simulink model "aes_impl_decrypt_smc"  (R2015b)
settings: Solver=FixedStepDiscrete  SolverMode=SingleTasking  StartTime=0.0  StopTime=1000e-6  RelTol=1e-3
undefined symbols (not defined in the file): a, b, input_sample_rate
libraries: shlslibv1 x3018
(part 9 of 20)

== system aes_impl_decrypt_smc/Round6/Subsystem8/Subsystem2 ==
  In1 : Inport
  In2 : Inport  Port=2
  In3 : Inport  Port=3
  In4 : Inport  Port=4
  Mixcolumn : Subsystem
  Mixcolumn1 : Subsystem
  Mixcolumn2 : Subsystem
  Mixcolumn3 : Subsystem
  Out1 : Outport
  Out2 : Outport  Port=2
  Out3 : Outport  Port=3
  Out4 : Outport  Port=4
  wires:
  Mixcolumn/1(Out1) -> Out1/1
  In4/1 -> Mixcolumn/4(In4), Mixcolumn1/4(In4), Mixcolumn2/4(In4), Mixcolumn3/4(In4)
  Mixcolumn2/1(Out1) -> Out3/1
  Mixcolumn1/1(Out1) -> Out2/1
  In2/1 -> Mixcolumn/2(In2), Mixcolumn1/2(In2), Mixcolumn3/2(In2), Mixcolumn2/2(In2)
  In1/1 -> Mixcolumn2/1(In1), Mixcolumn3/1(In1), Mixcolumn1/1(In1), Mixcolumn/1(In1)
  In3/1 -> Mixcolumn/3(In3), Mixcolumn1/3(In3), Mixcolumn3/3(In3), Mixcolumn2/3(In3)
  Mixcolumn3/1(Out1) -> Out4/1

== system aes_impl_decrypt_smc/Round6/Subsystem8/Subsystem3 ==
  In1 : Inport
  In2 : Inport  Port=2
  In3 : Inport  Port=3
  In4 : Inport  Port=4
  Mixcolumn : Subsystem
  Mixcolumn1 : Subsystem
  Mixcolumn2 : Subsystem
  Mixcolumn3 : Subsystem
  Out1 : Outport
  Out2 : Outport  Port=2
  Out3 : Outport  Port=3
  Out4 : Outport  Port=4
  wires:
  Mixcolumn/1(Out1) -> Out1/1
  In4/1 -> Mixcolumn/4(In4), Mixcolumn1/4(In4), Mixcolumn2/4(In4), Mixcolumn3/4(In4)
  Mixcolumn2/1(Out1) -> Out3/1
  Mixcolumn1/1(Out1) -> Out2/1
  In2/1 -> Mixcolumn/2(In2), Mixcolumn1/2(In2), Mixcolumn3/2(In2), Mixcolumn2/2(In2)
  In1/1 -> Mixcolumn2/1(In1), Mixcolumn3/1(In1), Mixcolumn1/1(In1), Mixcolumn/1(In1)
  In3/1 -> Mixcolumn/3(In3), Mixcolumn1/3(In3), Mixcolumn3/3(In3), Mixcolumn2/3(In3)
  Mixcolumn3/1(Out1) -> Out4/1

== system aes_impl_decrypt_smc/Round6/Subsystem8/Subsystem4 ==
  In1 : Inport
  In2 : Inport  Port=2
  In3 : Inport  Port=3
  In4 : Inport  Port=4
  ROM{1..4} (4 alike) : shlslibv1/Memories/ROM  syn_rom_vec=sbox  syn_rom_auto_wl=on  syn_out_wl=8  syn_out_fl=0  syn_out_dt=unsigned  syn_out_sat=on  syn_out_rnd=on  syn_en_port=off  synBlockType=primitive  synLatency=1  synBlockId=62  syn_dual_port=off
  Out1 : Outport
  Out2 : Outport  Port=2
  Out3 : Outport  Port=3
  Out4 : Outport  Port=4
  wires:
  In1/1 -> ROM4/1
  In4/1 -> ROM3/1
  In3/1 -> ROM2/1
  ROM4/1 -> Out1/1
  ROM1/1 -> Out2/1
  ROM2/1 -> Out3/1
  ROM3/1 -> Out4/1
  In2/1 -> ROM1/1

== system aes_impl_decrypt_smc/Round6/Subsystem8/Subsystem5 ==
  In1 : Inport
  In2 : Inport  Port=2
  In3 : Inport  Port=3
  In4 : Inport  Port=4
  ROM{1..4} (4 alike) : shlslibv1/Memories/ROM  syn_rom_vec=sbox  syn_rom_auto_wl=on  syn_out_wl=8  syn_out_fl=0  syn_out_dt=unsigned  syn_out_sat=on  syn_out_rnd=on  syn_en_port=off  synBlockType=primitive  synLatency=1  synBlockId=62  syn_dual_port=off
  Out1 : Outport
  Out2 : Outport  Port=2
  Out3 : Outport  Port=3
  Out4 : Outport  Port=4
  wires:
  In1/1 -> ROM4/1
  In4/1 -> ROM3/1
  In3/1 -> ROM2/1
  ROM4/1 -> Out1/1
  ROM1/1 -> Out2/1
  ROM2/1 -> Out3/1
  ROM3/1 -> Out4/1
  In2/1 -> ROM1/1

== system aes_impl_decrypt_smc/Round6/Subsystem8/Subsystem6 ==
  In1 : Inport
  In2 : Inport  Port=2
  In3 : Inport  Port=3
  In4 : Inport  Port=4
  ROM{1..4} (4 alike) : shlslibv1/Memories/ROM  syn_rom_vec=sbox  syn_rom_auto_wl=on  syn_out_wl=8  syn_out_fl=0  syn_out_dt=unsigned  syn_out_sat=on  syn_out_rnd=on  syn_en_port=off  synBlockType=primitive  synLatency=1  synBlockId=62  syn_dual_port=off
  Out1 : Outport
  Out2 : Outport  Port=2
  Out3 : Outport  Port=3
  Out4 : Outport  Port=4
  wires:
  In1/1 -> ROM4/1
  In4/1 -> ROM3/1
  In3/1 -> ROM2/1
  ROM4/1 -> Out1/1
  ROM1/1 -> Out2/1
  ROM2/1 -> Out3/1
  ROM3/1 -> Out4/1
  In2/1 -> ROM1/1

== system aes_impl_decrypt_smc/Round6/Subsystem8/Subsystem7 ==
  In1 : Inport
  In2 : Inport  Port=2
  In3 : Inport  Port=3
  In4 : Inport  Port=4
  ROM{1..4} (4 alike) : shlslibv1/Memories/ROM  syn_rom_vec=sbox  syn_rom_auto_wl=on  syn_out_wl=8  syn_out_fl=0  syn_out_dt=unsigned  syn_out_sat=on  syn_out_rnd=on  syn_en_port=off  synBlockType=primitive  synLatency=1  synBlockId=62  syn_dual_port=off
  Out1 : Outport
  Out2 : Outport  Port=2
  Out3 : Outport  Port=3
  Out4 : Outport  Port=4
  wires:
  In1/1 -> ROM4/1
  In4/1 -> ROM3/1
  In3/1 -> ROM2/1
  ROM4/1 -> Out1/1
  ROM1/1 -> Out2/1
  ROM2/1 -> Out3/1
  ROM3/1 -> Out4/1
  In2/1 -> ROM1/1

== system aes_impl_decrypt_smc/Round7/Key1/Keygen1 ==
  In1 : Inport
  In2 : Inport  Port=2
  In3 : Inport  Port=3
  In4 : Inport  Port=4
  In5 : Inport  Port=5
  In6 : Inport  Port=6
  In7 : Inport  Port=7
  In8 : Inport  Port=8
  Binary Logic{,1..7} (8 alike) : shlslibv1/Math Functions/Binary Logic  syn_binlog_exp=a^b  synBlockType=primitive  synLatency=0  synBlockId=13
  Constant1 : shlslibv1/Sources/Constant  syn_cst_val=0  syn_cst_format=Specify  syn_cst_wl=8  syn_cst_fl=0  syn_cst_dt=unsigned  syn_cst_rnd=on  syn_cst_st=-1  synBlockType=primitive  synLatency=0  synBlockId=15
  Constant2 : shlslibv1/Sources/Constant  syn_cst_val=0  syn_cst_format=Specify  syn_cst_wl=8  syn_cst_fl=0  syn_cst_dt=unsigned  syn_cst_rnd=on  syn_cst_st=-1  synBlockType=primitive  synLatency=0  synBlockId=15
  Constant3 : shlslibv1/Sources/Constant  syn_cst_val=0  syn_cst_format=Specify  syn_cst_wl=8  syn_cst_fl=0  syn_cst_dt=unsigned  syn_cst_rnd=on  syn_cst_st=-1  synBlockType=primitive  synLatency=0  synBlockId=15
  Constant4 : shlslibv1/Sources/Constant  syn_cst_val=64  syn_cst_format=Specify  syn_cst_wl=8  syn_cst_fl=0  syn_cst_dt=unsigned  syn_cst_rnd=on  syn_cst_st=-1  synBlockType=primitive  synLatency=0  synBlockId=15
  Subsystem4 : Subsystem
  Out1 : Outport
  Out2 : Outport  Port=2
  Out3 : Outport  Port=3
  Out4 : Outport  Port=4
  wires:
  Constant1/1 -> Binary Logic3/2
  Binary Logic3/1 -> Out2/1
  Binary Logic5/1 -> Out3/1
  Binary Logic2/1 -> Out1/1
  Constant3/1 -> Binary Logic7/2
  Binary Logic7/1 -> Out4/1
  Constant2/1 -> Binary Logic5/2
  Subsystem4/3(Out3) -> Binary Logic4/2
  In7/1 -> Subsystem4/2(In2)
  In6/1 -> Subsystem4/1(In1)
  Subsystem4/4(Out4) -> Binary Logic6/2
  Subsystem4/2(Out2) -> Binary Logic1/2
  Subsystem4/1(Out1) -> Binary Logic/2
  In8/1 -> Subsystem4/3(In3)
  In5/1 -> Subsystem4/4(In4)
  In1/1 -> Binary Logic/1
  In2/1 -> Binary Logic1/1
  In3/1 -> Binary Logic4/1
  In4/1 -> Binary Logic6/1
  Constant4/1 -> Binary Logic2/2
  Binary Logic/1 -> Binary Logic2/1
  Binary Logic1/1 -> Binary Logic3/1
  Binary Logic4/1 -> Binary Logic5/1
  Binary Logic6/1 -> Binary Logic7/1

== system aes_impl_decrypt_smc/Round7/Key1/Keygen2 ==
  In1 : Inport
  In2 : Inport  Port=2
  In3 : Inport  Port=3
  In4 : Inport  Port=4
  In5 : Inport  Port=5
  In6 : Inport  Port=6
  In7 : Inport  Port=7
  In8 : Inport  Port=8
  Binary Logic{,1..3} (4 alike) : shlslibv1/Math Functions/Binary Logic  syn_binlog_exp=a^b  synBlockType=primitive  synLatency=0  synBlockId=13
  Out1 : Outport
  Out2 : Outport  Port=2
  Out3 : Outport  Port=3
  Out4 : Outport  Port=4
  wires:
  In6/1 -> Binary Logic1/2
  In2/1 -> Binary Logic1/1
  Binary Logic2/1 -> Out3/1
  In7/1 -> Binary Logic2/2
  In8/1 -> Binary Logic3/2
  Binary Logic1/1 -> Out2/1
  In3/1 -> Binary Logic2/1
  In4/1 -> Binary Logic3/1
  Binary Logic3/1 -> Out4/1
  In1/1 -> Binary Logic/1
  In5/1 -> Binary Logic/2
  Binary Logic/1 -> Out1/1

== system aes_impl_decrypt_smc/Round7/Key1/Keygen3 ==
  In1 : Inport
  In2 : Inport  Port=2
  In3 : Inport  Port=3
  In4 : Inport  Port=4
  In5 : Inport  Port=5
  In6 : Inport  Port=6
  In7 : Inport  Port=7
  In8 : Inport  Port=8
  Binary Logic{,1..3} (4 alike) : shlslibv1/Math Functions/Binary Logic  syn_binlog_exp=a^b  synBlockType=primitive  synLatency=0  synBlockId=13
  Out1 : Outport
  Out2 : Outport  Port=2
  Out3 : Outport  Port=3
  Out4 : Outport  Port=4
  wires:
  In6/1 -> Binary Logic1/2
  In2/1 -> Binary Logic1/1
  Binary Logic2/1 -> Out3/1
  In7/1 -> Binary Logic2/2
  In8/1 -> Binary Logic3/2
  Binary Logic1/1 -> Out2/1
  In3/1 -> Binary Logic2/1
  In4/1 -> Binary Logic3/1
  Binary Logic3/1 -> Out4/1
  In1/1 -> Binary Logic/1
  In5/1 -> Binary Logic/2
  Binary Logic/1 -> Out1/1

== system aes_impl_decrypt_smc/Round7/Key1/Keygen4 ==
  In1 : Inport
  In2 : Inport  Port=2
  In3 : Inport  Port=3
  In4 : Inport  Port=4
  In5 : Inport  Port=5
  In6 : Inport  Port=6
  In7 : Inport  Port=7
  In8 : Inport  Port=8
  Binary Logic{,1..3} (4 alike) : shlslibv1/Math Functions/Binary Logic  syn_binlog_exp=a^b  synBlockType=primitive  synLatency=0  synBlockId=13
  Out1 : Outport
  Out2 : Outport  Port=2
  Out3 : Outport  Port=3
  Out4 : Outport  Port=4
  wires:
  In6/1 -> Binary Logic1/2
  In2/1 -> Binary Logic1/1
  Binary Logic2/1 -> Out3/1
  In7/1 -> Binary Logic2/2
  In8/1 -> Binary Logic3/2
  Binary Logic1/1 -> Out2/1
  In3/1 -> Binary Logic2/1
  In4/1 -> Binary Logic3/1
  Binary Logic3/1 -> Out4/1
  In1/1 -> Binary Logic/1
  In5/1 -> Binary Logic/2
  Binary Logic/1 -> Out1/1

== system aes_impl_decrypt_smc/Round7/Subsystem8/Subsystem ==
  In1 : Inport
  In2 : Inport  Port=2
  In3 : Inport  Port=3
  In4 : Inport  Port=4
  Mixcolumn : Subsystem
  Mixcolumn1 : Subsystem
  Mixcolumn2 : Subsystem
  Mixcolumn3 : Subsystem
  Out1 : Outport
  Out2 : Outport  Port=2
  Out3 : Outport  Port=3
  Out4 : Outport  Port=4
  wires:
  Mixcolumn/1(Out1) -> Out1/1
  In4/1 -> Mixcolumn/4(In4), Mixcolumn1/4(In4), Mixcolumn2/4(In4), Mixcolumn3/4(In4)
  Mixcolumn2/1(Out1) -> Out3/1
  Mixcolumn1/1(Out1) -> Out2/1
  In2/1 -> Mixcolumn/2(In2), Mixcolumn1/2(In2), Mixcolumn3/2(In2), Mixcolumn2/2(In2)
  In1/1 -> Mixcolumn2/1(In1), Mixcolumn3/1(In1), Mixcolumn1/1(In1), Mixcolumn/1(In1)
  In3/1 -> Mixcolumn/3(In3), Mixcolumn1/3(In3), Mixcolumn3/3(In3), Mixcolumn2/3(In3)
  Mixcolumn3/1(Out1) -> Out4/1

== system aes_impl_decrypt_smc/Round7/Subsystem8/Subsystem1 ==
  In1 : Inport
  In2 : Inport  Port=2
  In3 : Inport  Port=3
  In4 : Inport  Port=4
  Mixcolumn : Subsystem
  Mixcolumn1 : Subsystem
  Mixcolumn2 : Subsystem
  Mixcolumn3 : Subsystem
  Out1 : Outport
  Out2 : Outport  Port=2
  Out3 : Outport  Port=3
  Out4 : Outport  Port=4
  wires:
  Mixcolumn/1(Out1) -> Out1/1
  In4/1 -> Mixcolumn/4(In4), Mixcolumn1/4(In4), Mixcolumn2/4(In4), Mixcolumn3/4(In4)
  Mixcolumn2/1(Out1) -> Out3/1
  Mixcolumn1/1(Out1) -> Out2/1
  In2/1 -> Mixcolumn/2(In2), Mixcolumn1/2(In2), Mixcolumn3/2(In2), Mixcolumn2/2(In2)
  In1/1 -> Mixcolumn2/1(In1), Mixcolumn3/1(In1), Mixcolumn1/1(In1), Mixcolumn/1(In1)
  In3/1 -> Mixcolumn/3(In3), Mixcolumn1/3(In3), Mixcolumn3/3(In3), Mixcolumn2/3(In3)
  Mixcolumn3/1(Out1) -> Out4/1

== system aes_impl_decrypt_smc/Round7/Subsystem8/Subsystem2 ==
  In1 : Inport
  In2 : Inport  Port=2
  In3 : Inport  Port=3
  In4 : Inport  Port=4
  Mixcolumn : Subsystem
  Mixcolumn1 : Subsystem
  Mixcolumn2 : Subsystem
  Mixcolumn3 : Subsystem
  Out1 : Outport
  Out2 : Outport  Port=2
  Out3 : Outport  Port=3
  Out4 : Outport  Port=4
  wires:
  Mixcolumn/1(Out1) -> Out1/1
  In4/1 -> Mixcolumn/4(In4), Mixcolumn1/4(In4), Mixcolumn2/4(In4), Mixcolumn3/4(In4)
  Mixcolumn2/1(Out1) -> Out3/1
  Mixcolumn1/1(Out1) -> Out2/1
  In2/1 -> Mixcolumn/2(In2), Mixcolumn1/2(In2), Mixcolumn3/2(In2), Mixcolumn2/2(In2)
  In1/1 -> Mixcolumn2/1(In1), Mixcolumn3/1(In1), Mixcolumn1/1(In1), Mixcolumn/1(In1)
  In3/1 -> Mixcolumn/3(In3), Mixcolumn1/3(In3), Mixcolumn3/3(In3), Mixcolumn2/3(In3)
  Mixcolumn3/1(Out1) -> Out4/1

== system aes_impl_decrypt_smc/Round7/Subsystem8/Subsystem3 ==
  In1 : Inport
  In2 : Inport  Port=2
  In3 : Inport  Port=3
  In4 : Inport  Port=4
  Mixcolumn : Subsystem
  Mixcolumn1 : Subsystem
  Mixcolumn2 : Subsystem
  Mixcolumn3 : Subsystem
  Out1 : Outport
  Out2 : Outport  Port=2
  Out3 : Outport  Port=3
  Out4 : Outport  Port=4
  wires:
  Mixcolumn/1(Out1) -> Out1/1
  In4/1 -> Mixcolumn/4(In4), Mixcolumn1/4(In4), Mixcolumn2/4(In4), Mixcolumn3/4(In4)
  Mixcolumn2/1(Out1) -> Out3/1
  Mixcolumn1/1(Out1) -> Out2/1
  In2/1 -> Mixcolumn/2(In2), Mixcolumn1/2(In2), Mixcolumn3/2(In2), Mixcolumn2/2(In2)
  In1/1 -> Mixcolumn2/1(In1), Mixcolumn3/1(In1), Mixcolumn1/1(In1), Mixcolumn/1(In1)
  In3/1 -> Mixcolumn/3(In3), Mixcolumn1/3(In3), Mixcolumn3/3(In3), Mixcolumn2/3(In3)
  Mixcolumn3/1(Out1) -> Out4/1

== system aes_impl_decrypt_smc/Round7/Subsystem8/Subsystem4 ==
  In1 : Inport
  In2 : Inport  Port=2
  In3 : Inport  Port=3
  In4 : Inport  Port=4
  ROM{1..4} (4 alike) : shlslibv1/Memories/ROM  syn_rom_vec=sbox  syn_rom_auto_wl=on  syn_out_wl=8  syn_out_fl=0  syn_out_dt=unsigned  syn_out_sat=on  syn_out_rnd=on  syn_en_port=off  synBlockType=primitive  synLatency=1  synBlockId=62  syn_dual_port=off
  Out1 : Outport
  Out2 : Outport  Port=2
  Out3 : Outport  Port=3
  Out4 : Outport  Port=4
  wires:
  In1/1 -> ROM4/1
  In4/1 -> ROM3/1
  In3/1 -> ROM2/1
  ROM4/1 -> Out1/1
  ROM1/1 -> Out2/1
  ROM2/1 -> Out3/1
  ROM3/1 -> Out4/1
  In2/1 -> ROM1/1

== system aes_impl_decrypt_smc/Round7/Subsystem8/Subsystem5 ==
  In1 : Inport
  In2 : Inport  Port=2
  In3 : Inport  Port=3
  In4 : Inport  Port=4
  ROM{1..4} (4 alike) : shlslibv1/Memories/ROM  syn_rom_vec=sbox  syn_rom_auto_wl=on  syn_out_wl=8  syn_out_fl=0  syn_out_dt=unsigned  syn_out_sat=on  syn_out_rnd=on  syn_en_port=off  synBlockType=primitive  synLatency=1  synBlockId=62  syn_dual_port=off
  Out1 : Outport
  Out2 : Outport  Port=2
  Out3 : Outport  Port=3
  Out4 : Outport  Port=4
  wires:
  In1/1 -> ROM4/1
  In4/1 -> ROM3/1
  In3/1 -> ROM2/1
  ROM4/1 -> Out1/1
  ROM1/1 -> Out2/1
  ROM2/1 -> Out3/1
  ROM3/1 -> Out4/1
  In2/1 -> ROM1/1

== system aes_impl_decrypt_smc/Round7/Subsystem8/Subsystem6 ==
  In1 : Inport
  In2 : Inport  Port=2
  In3 : Inport  Port=3
  In4 : Inport  Port=4
  ROM{1..4} (4 alike) : shlslibv1/Memories/ROM  syn_rom_vec=sbox  syn_rom_auto_wl=on  syn_out_wl=8  syn_out_fl=0  syn_out_dt=unsigned  syn_out_sat=on  syn_out_rnd=on  syn_en_port=off  synBlockType=primitive  synLatency=1  synBlockId=62  syn_dual_port=off
  Out1 : Outport
  Out2 : Outport  Port=2
  Out3 : Outport  Port=3
  Out4 : Outport  Port=4
  wires:
  In1/1 -> ROM4/1
  In4/1 -> ROM3/1
  In3/1 -> ROM2/1
  ROM4/1 -> Out1/1
  ROM1/1 -> Out2/1
  ROM2/1 -> Out3/1
  ROM3/1 -> Out4/1
  In2/1 -> ROM1/1

== system aes_impl_decrypt_smc/Round7/Subsystem8/Subsystem7 ==
  In1 : Inport
  In2 : Inport  Port=2
  In3 : Inport  Port=3
  In4 : Inport  Port=4
  ROM{1..4} (4 alike) : shlslibv1/Memories/ROM  syn_rom_vec=sbox  syn_rom_auto_wl=on  syn_out_wl=8  syn_out_fl=0  syn_out_dt=unsigned  syn_out_sat=on  syn_out_rnd=on  syn_en_port=off  synBlockType=primitive  synLatency=1  synBlockId=62  syn_dual_port=off
  Out1 : Outport
  Out2 : Outport  Port=2
  Out3 : Outport  Port=3
  Out4 : Outport  Port=4
  wires:
  In1/1 -> ROM4/1
  In4/1 -> ROM3/1
  In3/1 -> ROM2/1
  ROM4/1 -> Out1/1
  ROM1/1 -> Out2/1
  ROM2/1 -> Out3/1
  ROM3/1 -> Out4/1
  In2/1 -> ROM1/1

== system aes_impl_decrypt_smc/Round8/Key1/Keygen1 ==
  In1 : Inport
  In2 : Inport  Port=2
  In3 : Inport  Port=3
  In4 : Inport  Port=4
  In5 : Inport  Port=5
  In6 : Inport  Port=6
  In7 : Inport  Port=7
  In8 : Inport  Port=8
  Binary Logic{,1..7} (8 alike) : shlslibv1/Math Functions/Binary Logic  syn_binlog_exp=a^b  synBlockType=primitive  synLatency=0  synBlockId=13
  Constant1 : shlslibv1/Sources/Constant  syn_cst_val=0  syn_cst_format=Specify  syn_cst_wl=8  syn_cst_fl=0  syn_cst_dt=unsigned  syn_cst_rnd=on  syn_cst_st=-1  synBlockType=primitive  synLatency=0  synBlockId=15
  Constant2 : shlslibv1/Sources/Constant  syn_cst_val=0  syn_cst_format=Specify  syn_cst_wl=8  syn_cst_fl=0  syn_cst_dt=unsigned  syn_cst_rnd=on  syn_cst_st=-1  synBlockType=primitive  synLatency=0  synBlockId=15
  Constant3 : shlslibv1/Sources/Constant  syn_cst_val=0  syn_cst_format=Specify  syn_cst_wl=8  syn_cst_fl=0  syn_cst_dt=unsigned  syn_cst_rnd=on  syn_cst_st=-1  synBlockType=primitive  synLatency=0  synBlockId=15
  Constant4 : shlslibv1/Sources/Constant  syn_cst_val=128  syn_cst_format=Specify  syn_cst_wl=8  syn_cst_fl=0  syn_cst_dt=unsigned  syn_cst_rnd=on  syn_cst_st=-1  synBlockType=primitive  synLatency=0  synBlockId=15
  Subsystem4 : Subsystem
  Out1 : Outport
  Out2 : Outport  Port=2
  Out3 : Outport  Port=3
  Out4 : Outport  Port=4
  wires:
  Constant1/1 -> Binary Logic3/2
  Binary Logic3/1 -> Out2/1
  Binary Logic5/1 -> Out3/1
  Binary Logic2/1 -> Out1/1
  Constant3/1 -> Binary Logic7/2
  Binary Logic7/1 -> Out4/1
  Constant2/1 -> Binary Logic5/2
  Subsystem4/3(Out3) -> Binary Logic4/2
  In7/1 -> Subsystem4/2(In2)
  In6/1 -> Subsystem4/1(In1)
  Subsystem4/4(Out4) -> Binary Logic6/2
  Subsystem4/2(Out2) -> Binary Logic1/2
  Subsystem4/1(Out1) -> Binary Logic/2
  In8/1 -> Subsystem4/3(In3)
  In5/1 -> Subsystem4/4(In4)
  In1/1 -> Binary Logic/1
  In2/1 -> Binary Logic1/1
  In3/1 -> Binary Logic4/1
  In4/1 -> Binary Logic6/1
  Constant4/1 -> Binary Logic2/2
  Binary Logic/1 -> Binary Logic2/1
  Binary Logic1/1 -> Binary Logic3/1
  Binary Logic4/1 -> Binary Logic5/1
  Binary Logic6/1 -> Binary Logic7/1

== system aes_impl_decrypt_smc/Round8/Key1/Keygen2 ==
  In1 : Inport
  In2 : Inport  Port=2
  In3 : Inport  Port=3
  In4 : Inport  Port=4
  In5 : Inport  Port=5
  In6 : Inport  Port=6
  In7 : Inport  Port=7
  In8 : Inport  Port=8
  Binary Logic{,1..3} (4 alike) : shlslibv1/Math Functions/Binary Logic  syn_binlog_exp=a^b  synBlockType=primitive  synLatency=0  synBlockId=13
  Out1 : Outport
  Out2 : Outport  Port=2
  Out3 : Outport  Port=3
  Out4 : Outport  Port=4
  wires:
  In6/1 -> Binary Logic1/2
  In2/1 -> Binary Logic1/1
  Binary Logic2/1 -> Out3/1
  In7/1 -> Binary Logic2/2
  In8/1 -> Binary Logic3/2
  Binary Logic1/1 -> Out2/1
  In3/1 -> Binary Logic2/1
  In4/1 -> Binary Logic3/1
  Binary Logic3/1 -> Out4/1
  In1/1 -> Binary Logic/1
  In5/1 -> Binary Logic/2
  Binary Logic/1 -> Out1/1

== system aes_impl_decrypt_smc/Round8/Key1/Keygen3 ==
  In1 : Inport
  In2 : Inport  Port=2
  In3 : Inport  Port=3
  In4 : Inport  Port=4
  In5 : Inport  Port=5
  In6 : Inport  Port=6
  In7 : Inport  Port=7
  In8 : Inport  Port=8
  Binary Logic{,1..3} (4 alike) : shlslibv1/Math Functions/Binary Logic  syn_binlog_exp=a^b  synBlockType=primitive  synLatency=0  synBlockId=13
  Out1 : Outport
  Out2 : Outport  Port=2
  Out3 : Outport  Port=3
  Out4 : Outport  Port=4
  wires:
  In6/1 -> Binary Logic1/2
  In2/1 -> Binary Logic1/1
  Binary Logic2/1 -> Out3/1
  In7/1 -> Binary Logic2/2
  In8/1 -> Binary Logic3/2
  Binary Logic1/1 -> Out2/1
  In3/1 -> Binary Logic2/1
  In4/1 -> Binary Logic3/1
  Binary Logic3/1 -> Out4/1
  In1/1 -> Binary Logic/1
  In5/1 -> Binary Logic/2
  Binary Logic/1 -> Out1/1

== system aes_impl_decrypt_smc/Round8/Key1/Keygen4 ==
  In1 : Inport
  In2 : Inport  Port=2
  In3 : Inport  Port=3
  In4 : Inport  Port=4
  In5 : Inport  Port=5
  In6 : Inport  Port=6
  In7 : Inport  Port=7
  In8 : Inport  Port=8
  Binary Logic{,1..3} (4 alike) : shlslibv1/Math Functions/Binary Logic  syn_binlog_exp=a^b  synBlockType=primitive  synLatency=0  synBlockId=13
  Out1 : Outport
  Out2 : Outport  Port=2
  Out3 : Outport  Port=3
  Out4 : Outport  Port=4
  wires:
  In6/1 -> Binary Logic1/2
  In2/1 -> Binary Logic1/1
  Binary Logic2/1 -> Out3/1
  In7/1 -> Binary Logic2/2
  In8/1 -> Binary Logic3/2
  Binary Logic1/1 -> Out2/1
  In3/1 -> Binary Logic2/1
  In4/1 -> Binary Logic3/1
  Binary Logic3/1 -> Out4/1
  In1/1 -> Binary Logic/1
  In5/1 -> Binary Logic/2
  Binary Logic/1 -> Out1/1

== system aes_impl_decrypt_smc/Round8/Subsystem8/Subsystem ==
  In1 : Inport
  In2 : Inport  Port=2
  In3 : Inport  Port=3
  In4 : Inport  Port=4
  Mixcolumn : Subsystem
  Mixcolumn1 : Subsystem
  Mixcolumn2 : Subsystem
  Mixcolumn3 : Subsystem
  Out1 : Outport
  Out2 : Outport  Port=2
  Out3 : Outport  Port=3
  Out4 : Outport  Port=4
  wires:
  Mixcolumn/1(Out1) -> Out1/1
  In4/1 -> Mixcolumn/4(In4), Mixcolumn1/4(In4), Mixcolumn2/4(In4), Mixcolumn3/4(In4)
  Mixcolumn2/1(Out1) -> Out3/1
  Mixcolumn1/1(Out1) -> Out2/1
  In2/1 -> Mixcolumn/2(In2), Mixcolumn1/2(In2), Mixcolumn3/2(In2), Mixcolumn2/2(In2)
  In1/1 -> Mixcolumn2/1(In1), Mixcolumn3/1(In1), Mixcolumn1/1(In1), Mixcolumn/1(In1)
  In3/1 -> Mixcolumn/3(In3), Mixcolumn1/3(In3), Mixcolumn3/3(In3), Mixcolumn2/3(In3)
  Mixcolumn3/1(Out1) -> Out4/1

== system aes_impl_decrypt_smc/Round8/Subsystem8/Subsystem1 ==
  In1 : Inport
  In2 : Inport  Port=2
  In3 : Inport  Port=3
  In4 : Inport  Port=4
  Mixcolumn : Subsystem
  Mixcolumn1 : Subsystem
  Mixcolumn2 : Subsystem
  Mixcolumn3 : Subsystem
  Out1 : Outport
  Out2 : Outport  Port=2
  Out3 : Outport  Port=3
  Out4 : Outport  Port=4
  wires:
  Mixcolumn/1(Out1) -> Out1/1
  In4/1 -> Mixcolumn/4(In4), Mixcolumn1/4(In4), Mixcolumn2/4(In4), Mixcolumn3/4(In4)
  Mixcolumn2/1(Out1) -> Out3/1
  Mixcolumn1/1(Out1) -> Out2/1
  In2/1 -> Mixcolumn/2(In2), Mixcolumn1/2(In2), Mixcolumn3/2(In2), Mixcolumn2/2(In2)
  In1/1 -> Mixcolumn2/1(In1), Mixcolumn3/1(In1), Mixcolumn1/1(In1), Mixcolumn/1(In1)
  In3/1 -> Mixcolumn/3(In3), Mixcolumn1/3(In3), Mixcolumn3/3(In3), Mixcolumn2/3(In3)
  Mixcolumn3/1(Out1) -> Out4/1

== system aes_impl_decrypt_smc/Round8/Subsystem8/Subsystem2 ==
  In1 : Inport
  In2 : Inport  Port=2
  In3 : Inport  Port=3
  In4 : Inport  Port=4
  Mixcolumn : Subsystem
  Mixcolumn1 : Subsystem
  Mixcolumn2 : Subsystem
  Mixcolumn3 : Subsystem
  Out1 : Outport
  Out2 : Outport  Port=2
  Out3 : Outport  Port=3
  Out4 : Outport  Port=4
  wires:
  Mixcolumn/1(Out1) -> Out1/1
  In4/1 -> Mixcolumn/4(In4), Mixcolumn1/4(In4), Mixcolumn2/4(In4), Mixcolumn3/4(In4)
  Mixcolumn2/1(Out1) -> Out3/1
  Mixcolumn1/1(Out1) -> Out2/1
  In2/1 -> Mixcolumn/2(In2), Mixcolumn1/2(In2), Mixcolumn3/2(In2), Mixcolumn2/2(In2)
  In1/1 -> Mixcolumn2/1(In1), Mixcolumn3/1(In1), Mixcolumn1/1(In1), Mixcolumn/1(In1)
  In3/1 -> Mixcolumn/3(In3), Mixcolumn1/3(In3), Mixcolumn3/3(In3), Mixcolumn2/3(In3)
  Mixcolumn3/1(Out1) -> Out4/1

== system aes_impl_decrypt_smc/Round8/Subsystem8/Subsystem3 ==
  In1 : Inport
  In2 : Inport  Port=2
  In3 : Inport  Port=3
  In4 : Inport  Port=4
  Mixcolumn : Subsystem
  Mixcolumn1 : Subsystem
  Mixcolumn2 : Subsystem
  Mixcolumn3 : Subsystem
  Out1 : Outport
  Out2 : Outport  Port=2
  Out3 : Outport  Port=3
  Out4 : Outport  Port=4
  wires:
  Mixcolumn/1(Out1) -> Out1/1
  In4/1 -> Mixcolumn/4(In4), Mixcolumn1/4(In4), Mixcolumn2/4(In4), Mixcolumn3/4(In4)
  Mixcolumn2/1(Out1) -> Out3/1
  Mixcolumn1/1(Out1) -> Out2/1
  In2/1 -> Mixcolumn/2(In2), Mixcolumn1/2(In2), Mixcolumn3/2(In2), Mixcolumn2/2(In2)
  In1/1 -> Mixcolumn2/1(In1), Mixcolumn3/1(In1), Mixcolumn1/1(In1), Mixcolumn/1(In1)
  In3/1 -> Mixcolumn/3(In3), Mixcolumn1/3(In3), Mixcolumn3/3(In3), Mixcolumn2/3(In3)
  Mixcolumn3/1(Out1) -> Out4/1

== system aes_impl_decrypt_smc/Round8/Subsystem8/Subsystem4 ==
  In1 : Inport
  In2 : Inport  Port=2
  In3 : Inport  Port=3
  In4 : Inport  Port=4
  ROM{1..4} (4 alike) : shlslibv1/Memories/ROM  syn_rom_vec=sbox  syn_rom_auto_wl=on  syn_out_wl=8  syn_out_fl=0  syn_out_dt=unsigned  syn_out_sat=on  syn_out_rnd=on  syn_en_port=off  synBlockType=primitive  synLatency=1  synBlockId=62  syn_dual_port=off
  Out1 : Outport
  Out2 : Outport  Port=2
  Out3 : Outport  Port=3
  Out4 : Outport  Port=4
  wires:
  In1/1 -> ROM4/1
  In4/1 -> ROM3/1
  In3/1 -> ROM2/1
  ROM4/1 -> Out1/1
  ROM1/1 -> Out2/1
  ROM2/1 -> Out3/1
  ROM3/1 -> Out4/1
  In2/1 -> ROM1/1

== system aes_impl_decrypt_smc/Round8/Subsystem8/Subsystem5 ==
  In1 : Inport
  In2 : Inport  Port=2
  In3 : Inport  Port=3
  In4 : Inport  Port=4
  ROM{1..4} (4 alike) : shlslibv1/Memories/ROM  syn_rom_vec=sbox  syn_rom_auto_wl=on  syn_out_wl=8  syn_out_fl=0  syn_out_dt=unsigned  syn_out_sat=on  syn_out_rnd=on  syn_en_port=off  synBlockType=primitive  synLatency=1  synBlockId=62  syn_dual_port=off
  Out1 : Outport
  Out2 : Outport  Port=2
  Out3 : Outport  Port=3
  Out4 : Outport  Port=4
  wires:
  In1/1 -> ROM4/1
  In4/1 -> ROM3/1
  In3/1 -> ROM2/1
  ROM4/1 -> Out1/1
  ROM1/1 -> Out2/1
  ROM2/1 -> Out3/1
  ROM3/1 -> Out4/1
  In2/1 -> ROM1/1

== system aes_impl_decrypt_smc/Round8/Subsystem8/Subsystem6 ==
  In1 : Inport
  In2 : Inport  Port=2
  In3 : Inport  Port=3
  In4 : Inport  Port=4
  ROM{1..4} (4 alike) : shlslibv1/Memories/ROM  syn_rom_vec=sbox  syn_rom_auto_wl=on  syn_out_wl=8  syn_out_fl=0  syn_out_dt=unsigned  syn_out_sat=on  syn_out_rnd=on  syn_en_port=off  synBlockType=primitive  synLatency=1  synBlockId=62  syn_dual_port=off
  Out1 : Outport
  Out2 : Outport  Port=2
  Out3 : Outport  Port=3
  Out4 : Outport  Port=4
  wires:
  In1/1 -> ROM4/1
  In4/1 -> ROM3/1
  In3/1 -> ROM2/1
  ROM4/1 -> Out1/1
  ROM1/1 -> Out2/1
  ROM2/1 -> Out3/1
  ROM3/1 -> Out4/1
  In2/1 -> ROM1/1

== system aes_impl_decrypt_smc/Round8/Subsystem8/Subsystem7 ==
  In1 : Inport
  In2 : Inport  Port=2
  In3 : Inport  Port=3
  In4 : Inport  Port=4
  ROM{1..4} (4 alike) : shlslibv1/Memories/ROM  syn_rom_vec=sbox  syn_rom_auto_wl=on  syn_out_wl=8  syn_out_fl=0  syn_out_dt=unsigned  syn_out_sat=on  syn_out_rnd=on  syn_en_port=off  synBlockType=primitive  synLatency=1  synBlockId=62  syn_dual_port=off
  Out1 : Outport
  Out2 : Outport  Port=2
  Out3 : Outport  Port=3
  Out4 : Outport  Port=4
  wires:
  In1/1 -> ROM4/1
  In4/1 -> ROM3/1
  In3/1 -> ROM2/1
  ROM4/1 -> Out1/1
  ROM1/1 -> Out2/1
  ROM2/1 -> Out3/1
  ROM3/1 -> Out4/1
  In2/1 -> ROM1/1

== system aes_impl_decrypt_smc/Round9/Key1/Keygen1 ==
  In1 : Inport
  In2 : Inport  Port=2
  In3 : Inport  Port=3
  In4 : Inport  Port=4
  In5 : Inport  Port=5
  In6 : Inport  Port=6
  In7 : Inport  Port=7
  In8 : Inport  Port=8
  Binary Logic{,1..7} (8 alike) : shlslibv1/Math Functions/Binary Logic  syn_binlog_exp=a^b  synBlockType=primitive  synLatency=0  synBlockId=13
  Constant1 : shlslibv1/Sources/Constant  syn_cst_val=0  syn_cst_format=Specify  syn_cst_wl=8  syn_cst_fl=0  syn_cst_dt=unsigned  syn_cst_rnd=on  syn_cst_st=-1  synBlockType=primitive  synLatency=0  synBlockId=15
  Constant2 : shlslibv1/Sources/Constant  syn_cst_val=0  syn_cst_format=Specify  syn_cst_wl=8  syn_cst_fl=0  syn_cst_dt=unsigned  syn_cst_rnd=on  syn_cst_st=-1  synBlockType=primitive  synLatency=0  synBlockId=15
  Constant3 : shlslibv1/Sources/Constant  syn_cst_val=0  syn_cst_format=Specify  syn_cst_wl=8  syn_cst_fl=0  syn_cst_dt=unsigned  syn_cst_rnd=on  syn_cst_st=-1  synBlockType=primitive  synLatency=0  synBlockId=15
  Constant4 : shlslibv1/Sources/Constant  syn_cst_val=27  syn_cst_format=Specify  syn_cst_wl=8  syn_cst_fl=0  syn_cst_dt=unsigned  syn_cst_rnd=on  syn_cst_st=-1  synBlockType=primitive  synLatency=0  synBlockId=15
  Subsystem4 : Subsystem
  Out1 : Outport
  Out2 : Outport  Port=2
  Out3 : Outport  Port=3
  Out4 : Outport  Port=4
  wires:
  Constant1/1 -> Binary Logic3/2
  Binary Logic3/1 -> Out2/1
  Binary Logic5/1 -> Out3/1
  Binary Logic2/1 -> Out1/1
  Constant3/1 -> Binary Logic7/2
  Binary Logic7/1 -> Out4/1
  Constant2/1 -> Binary Logic5/2
  Subsystem4/3(Out3) -> Binary Logic4/2
  In7/1 -> Subsystem4/2(In2)
  In6/1 -> Subsystem4/1(In1)
  Subsystem4/4(Out4) -> Binary Logic6/2
  Subsystem4/2(Out2) -> Binary Logic1/2
  Subsystem4/1(Out1) -> Binary Logic/2
  In8/1 -> Subsystem4/3(In3)
  In5/1 -> Subsystem4/4(In4)
  In1/1 -> Binary Logic/1
  In2/1 -> Binary Logic1/1
  In3/1 -> Binary Logic4/1
  In4/1 -> Binary Logic6/1
  Constant4/1 -> Binary Logic2/2
  Binary Logic/1 -> Binary Logic2/1
  Binary Logic1/1 -> Binary Logic3/1
  Binary Logic4/1 -> Binary Logic5/1
  Binary Logic6/1 -> Binary Logic7/1

== system aes_impl_decrypt_smc/Round9/Key1/Keygen2 ==
  In1 : Inport
  In2 : Inport  Port=2
  In3 : Inport  Port=3
  In4 : Inport  Port=4
  In5 : Inport  Port=5
  In6 : Inport  Port=6
  In7 : Inport  Port=7
  In8 : Inport  Port=8
  Binary Logic{,1..3} (4 alike) : shlslibv1/Math Functions/Binary Logic  syn_binlog_exp=a^b  synBlockType=primitive  synLatency=0  synBlockId=13
  Out1 : Outport
  Out2 : Outport  Port=2
  Out3 : Outport  Port=3
  Out4 : Outport  Port=4
  wires:
  In6/1 -> Binary Logic1/2
  In2/1 -> Binary Logic1/1
  Binary Logic2/1 -> Out3/1
  In7/1 -> Binary Logic2/2
  In8/1 -> Binary Logic3/2
  Binary Logic1/1 -> Out2/1
  In3/1 -> Binary Logic2/1
  In4/1 -> Binary Logic3/1
  Binary Logic3/1 -> Out4/1
  In1/1 -> Binary Logic/1
  In5/1 -> Binary Logic/2
  Binary Logic/1 -> Out1/1

== system aes_impl_decrypt_smc/Round9/Key1/Keygen3 ==
  In1 : Inport
  In2 : Inport  Port=2
  In3 : Inport  Port=3
  In4 : Inport  Port=4
  In5 : Inport  Port=5
  In6 : Inport  Port=6
  In7 : Inport  Port=7
  In8 : Inport  Port=8
  Binary Logic{,1..3} (4 alike) : shlslibv1/Math Functions/Binary Logic  syn_binlog_exp=a^b  synBlockType=primitive  synLatency=0  synBlockId=13
  Out1 : Outport
  Out2 : Outport  Port=2
  Out3 : Outport  Port=3
  Out4 : Outport  Port=4
  wires:
  In6/1 -> Binary Logic1/2
  In2/1 -> Binary Logic1/1
  Binary Logic2/1 -> Out3/1
  In7/1 -> Binary Logic2/2
  In8/1 -> Binary Logic3/2
  Binary Logic1/1 -> Out2/1
  In3/1 -> Binary Logic2/1
  In4/1 -> Binary Logic3/1
  Binary Logic3/1 -> Out4/1
  In1/1 -> Binary Logic/1
  In5/1 -> Binary Logic/2
  Binary Logic/1 -> Out1/1

== system aes_impl_decrypt_smc/Round9/Key1/Keygen4 ==
  In1 : Inport
  In2 : Inport  Port=2
  In3 : Inport  Port=3
  In4 : Inport  Port=4
  In5 : Inport  Port=5
  In6 : Inport  Port=6
  In7 : Inport  Port=7
  In8 : Inport  Port=8
  Binary Logic{,1..3} (4 alike) : shlslibv1/Math Functions/Binary Logic  syn_binlog_exp=a^b  synBlockType=primitive  synLatency=0  synBlockId=13
  Out1 : Outport
  Out2 : Outport  Port=2
  Out3 : Outport  Port=3
  Out4 : Outport  Port=4
  wires:
  In6/1 -> Binary Logic1/2
  In2/1 -> Binary Logic1/1
  Binary Logic2/1 -> Out3/1
  In7/1 -> Binary Logic2/2
  In8/1 -> Binary Logic3/2
  Binary Logic1/1 -> Out2/1
  In3/1 -> Binary Logic2/1
  In4/1 -> Binary Logic3/1
  Binary Logic3/1 -> Out4/1
  In1/1 -> Binary Logic/1
  In5/1 -> Binary Logic/2
  Binary Logic/1 -> Out1/1

== system aes_impl_decrypt_smc/Round9/Subsystem8/Subsystem ==
  In1 : Inport
  In2 : Inport  Port=2
  In3 : Inport  Port=3
  In4 : Inport  Port=4
  Mixcolumn : Subsystem
  Mixcolumn1 : Subsystem
  Mixcolumn2 : Subsystem
  Mixcolumn3 : Subsystem
  Out1 : Outport
  Out2 : Outport  Port=2
  Out3 : Outport  Port=3
  Out4 : Outport  Port=4
  wires:
  Mixcolumn/1(Out1) -> Out1/1
  In4/1 -> Mixcolumn/4(In4), Mixcolumn1/4(In4), Mixcolumn2/4(In4), Mixcolumn3/4(In4)
  Mixcolumn2/1(Out1) -> Out3/1
  Mixcolumn1/1(Out1) -> Out2/1
  In2/1 -> Mixcolumn/2(In2), Mixcolumn1/2(In2), Mixcolumn3/2(In2), Mixcolumn2/2(In2)
  In1/1 -> Mixcolumn2/1(In1), Mixcolumn3/1(In1), Mixcolumn1/1(In1), Mixcolumn/1(In1)
  In3/1 -> Mixcolumn/3(In3), Mixcolumn1/3(In3), Mixcolumn3/3(In3), Mixcolumn2/3(In3)
  Mixcolumn3/1(Out1) -> Out4/1

== system aes_impl_decrypt_smc/Round9/Subsystem8/Subsystem1 ==
  In1 : Inport
  In2 : Inport  Port=2
  In3 : Inport  Port=3
  In4 : Inport  Port=4
  Mixcolumn : Subsystem
  Mixcolumn1 : Subsystem
  Mixcolumn2 : Subsystem
  Mixcolumn3 : Subsystem
  Out1 : Outport
  Out2 : Outport  Port=2
  Out3 : Outport  Port=3
  Out4 : Outport  Port=4
  wires:
  Mixcolumn/1(Out1) -> Out1/1
  In4/1 -> Mixcolumn/4(In4), Mixcolumn1/4(In4), Mixcolumn2/4(In4), Mixcolumn3/4(In4)
  Mixcolumn2/1(Out1) -> Out3/1
  Mixcolumn1/1(Out1) -> Out2/1
  In2/1 -> Mixcolumn/2(In2), Mixcolumn1/2(In2), Mixcolumn3/2(In2), Mixcolumn2/2(In2)
  In1/1 -> Mixcolumn2/1(In1), Mixcolumn3/1(In1), Mixcolumn1/1(In1), Mixcolumn/1(In1)
  In3/1 -> Mixcolumn/3(In3), Mixcolumn1/3(In3), Mixcolumn3/3(In3), Mixcolumn2/3(In3)
  Mixcolumn3/1(Out1) -> Out4/1

== system aes_impl_decrypt_smc/Round9/Subsystem8/Subsystem2 ==
  In1 : Inport
  In2 : Inport  Port=2
  In3 : Inport  Port=3
  In4 : Inport  Port=4
  Mixcolumn : Subsystem
  Mixcolumn1 : Subsystem
  Mixcolumn2 : Subsystem
  Mixcolumn3 : Subsystem
  Out1 : Outport
  Out2 : Outport  Port=2
  Out3 : Outport  Port=3
  Out4 : Outport  Port=4
  wires:
  Mixcolumn/1(Out1) -> Out1/1
  In4/1 -> Mixcolumn/4(In4), Mixcolumn1/4(In4), Mixcolumn2/4(In4), Mixcolumn3/4(In4)
  Mixcolumn2/1(Out1) -> Out3/1
  Mixcolumn1/1(Out1) -> Out2/1
  In2/1 -> Mixcolumn/2(In2), Mixcolumn1/2(In2), Mixcolumn3/2(In2), Mixcolumn2/2(In2)
  In1/1 -> Mixcolumn2/1(In1), Mixcolumn3/1(In1), Mixcolumn1/1(In1), Mixcolumn/1(In1)
  In3/1 -> Mixcolumn/3(In3), Mixcolumn1/3(In3), Mixcolumn3/3(In3), Mixcolumn2/3(In3)
  Mixcolumn3/1(Out1) -> Out4/1

== system aes_impl_decrypt_smc/Round9/Subsystem8/Subsystem3 ==
  In1 : Inport
  In2 : Inport  Port=2
  In3 : Inport  Port=3
  In4 : Inport  Port=4
  Mixcolumn : Subsystem
  Mixcolumn1 : Subsystem
  Mixcolumn2 : Subsystem
  Mixcolumn3 : Subsystem
  Out1 : Outport
  Out2 : Outport  Port=2
  Out3 : Outport  Port=3
  Out4 : Outport  Port=4
  wires:
  Mixcolumn/1(Out1) -> Out1/1
  In4/1 -> Mixcolumn/4(In4), Mixcolumn1/4(In4), Mixcolumn2/4(In4), Mixcolumn3/4(In4)
  Mixcolumn2/1(Out1) -> Out3/1
  Mixcolumn1/1(Out1) -> Out2/1
  In2/1 -> Mixcolumn/2(In2), Mixcolumn1/2(In2), Mixcolumn3/2(In2), Mixcolumn2/2(In2)
  In1/1 -> Mixcolumn2/1(In1), Mixcolumn3/1(In1), Mixcolumn1/1(In1), Mixcolumn/1(In1)
  In3/1 -> Mixcolumn/3(In3), Mixcolumn1/3(In3), Mixcolumn3/3(In3), Mixcolumn2/3(In3)
  Mixcolumn3/1(Out1) -> Out4/1

== system aes_impl_decrypt_smc/Round9/Subsystem8/Subsystem4 ==
  In1 : Inport
  In2 : Inport  Port=2
  In3 : Inport  Port=3
  In4 : Inport  Port=4
  ROM{1..4} (4 alike) : shlslibv1/Memories/ROM  syn_rom_vec=sbox  syn_rom_auto_wl=on  syn_out_wl=8  syn_out_fl=0  syn_out_dt=unsigned  syn_out_sat=on  syn_out_rnd=on  syn_en_port=off  synBlockType=primitive  synLatency=1  synBlockId=62  syn_dual_port=off
  Out1 : Outport
  Out2 : Outport  Port=2
  Out3 : Outport  Port=3
  Out4 : Outport  Port=4
  wires:
  In1/1 -> ROM4/1
  In4/1 -> ROM3/1
  In3/1 -> ROM2/1
  ROM4/1 -> Out1/1
  ROM1/1 -> Out2/1
  ROM2/1 -> Out3/1
  ROM3/1 -> Out4/1
  In2/1 -> ROM1/1

== system aes_impl_decrypt_smc/Round9/Subsystem8/Subsystem5 ==
  In1 : Inport
  In2 : Inport  Port=2
  In3 : Inport  Port=3
  In4 : Inport  Port=4
  ROM{1..4} (4 alike) : shlslibv1/Memories/ROM  syn_rom_vec=sbox  syn_rom_auto_wl=on  syn_out_wl=8  syn_out_fl=0  syn_out_dt=unsigned  syn_out_sat=on  syn_out_rnd=on  syn_en_port=off  synBlockType=primitive  synLatency=1  synBlockId=62  syn_dual_port=off
  Out1 : Outport
  Out2 : Outport  Port=2
  Out3 : Outport  Port=3
  Out4 : Outport  Port=4
  wires:
  In1/1 -> ROM4/1
  In4/1 -> ROM3/1
  In3/1 -> ROM2/1
  ROM4/1 -> Out1/1
  ROM1/1 -> Out2/1
  ROM2/1 -> Out3/1
  ROM3/1 -> Out4/1
  In2/1 -> ROM1/1

== system aes_impl_decrypt_smc/Round9/Subsystem8/Subsystem6 ==
  In1 : Inport
  In2 : Inport  Port=2
  In3 : Inport  Port=3
  In4 : Inport  Port=4
  ROM{1..4} (4 alike) : shlslibv1/Memories/ROM  syn_rom_vec=sbox  syn_rom_auto_wl=on  syn_out_wl=8  syn_out_fl=0  syn_out_dt=unsigned  syn_out_sat=on  syn_out_rnd=on  syn_en_port=off  synBlockType=primitive  synLatency=1  synBlockId=62  syn_dual_port=off
  Out1 : Outport
  Out2 : Outport  Port=2
  Out3 : Outport  Port=3
  Out4 : Outport  Port=4
  wires:
  In1/1 -> ROM4/1
  In4/1 -> ROM3/1
  In3/1 -> ROM2/1
  ROM4/1 -> Out1/1
  ROM1/1 -> Out2/1
  ROM2/1 -> Out3/1
  ROM3/1 -> Out4/1
  In2/1 -> ROM1/1

== system aes_impl_decrypt_smc/Round9/Subsystem8/Subsystem7 ==
  In1 : Inport
  In2 : Inport  Port=2
  In3 : Inport  Port=3
  In4 : Inport  Port=4
  ROM{1..4} (4 alike) : shlslibv1/Memories/ROM  syn_rom_vec=sbox  syn_rom_auto_wl=on  syn_out_wl=8  syn_out_fl=0  syn_out_dt=unsigned  syn_out_sat=on  syn_out_rnd=on  syn_en_port=off  synBlockType=primitive  synLatency=1  synBlockId=62  syn_dual_port=off
  Out1 : Outport
  Out2 : Outport  Port=2
  Out3 : Outport  Port=3
  Out4 : Outport  Port=4
  wires:
  In1/1 -> ROM4/1
  In4/1 -> ROM3/1
  In3/1 -> ROM2/1
  ROM4/1 -> Out1/1
  ROM1/1 -> Out2/1
  ROM2/1 -> Out3/1
  ROM3/1 -> Out4/1
  In2/1 -> ROM1/1

== system aes_impl_decrypt_smc/Round1/Key1/Keygen1/Subsystem4 ==
  In1 : Inport
  In2 : Inport  Port=2
  In3 : Inport  Port=3
  In4 : Inport  Port=4
  ROM{1..4} (4 alike) : shlslibv1/Memories/ROM  syn_rom_vec=sbox  syn_rom_auto_wl=on  syn_out_wl=8  syn_out_fl=0  syn_out_dt=unsigned  syn_out_sat=on  syn_out_rnd=on  syn_en_port=off  synBlockType=primitive  synLatency=1  synBlockId=62  syn_dual_port=off
  Out1 : Outport
  Out2 : Outport  Port=2
  Out3 : Outport  Port=3
  Out4 : Outport  Port=4
  wires:
  In1/1 -> ROM4/1
  In4/1 -> ROM3/1
  In3/1 -> ROM2/1
  ROM4/1 -> Out1/1
  ROM1/1 -> Out2/1
  ROM2/1 -> Out3/1
  ROM3/1 -> Out4/1
  In2/1 -> ROM1/1

== system aes_impl_decrypt_smc/Round1/Subsystem8/Subsystem/Mixcolumn ==
  In1 : Inport
  In2 : Inport  Port=2
  In3 : Inport  Port=3
  In4 : Inport  Port=4
  Binary Logic : shlslibv1/Math Functions/Binary Logic  syn_binlog_exp=a^b  synBlockType=primitive  synLatency=0  synBlockId=13
  Binary Logic1 : shlslibv1/Math Functions/Binary Logic  syn_binlog_exp=a^b  synBlockType=primitive  synLatency=0  synBlockId=13
  Binary Logic2 : shlslibv1/Math Functions/Binary Logic  syn_binlog_exp=a^b  synBlockType=primitive  synLatency=0  synBlockId=13
  Display{,1..3,5} (5 alike) : Display
      settings: Format=hex (Stored Integer)
  Port Out : shlslibv1/Ports & Subsystems/Port Out  syn_capture=on  syn_register=on  synBlockType=port  synLatency=1  synBlockId=1
  multiplier2 : shlslibv1/Memories/ROM  syn_rom_vec=multiplier2  syn_rom_auto_wl=on  syn_out_wl=8  syn_out_fl=0  syn_out_dt=unsigned  syn_out_sat=on  syn_out_rnd=on  syn_en_port=off  synBlockType=primitive  synLatency=1  synBlockId=62  syn_dual_port=off
  multiplier3 : shlslibv1/Memories/ROM  syn_rom_vec=multiplier3  syn_rom_auto_wl=on  syn_out_wl=8  syn_out_fl=0  syn_out_dt=unsigned  syn_out_sat=on  syn_out_rnd=on  syn_en_port=off  synBlockType=primitive  synLatency=1  synBlockId=62  syn_dual_port=off
  Out1 : Outport
  wires:
  multiplier3/1 -> Binary Logic/2
  In2/1 -> Display1/1, multiplier3/1
  In4/1 -> Binary Logic1/2
  multiplier2/1 -> Binary Logic/1
  In3/1 -> Binary Logic1/1
  Binary Logic2/1 -> Port Out/1, Out1/1
  Port Out/1 -> Display5/1
  Binary Logic/1 -> Display2/1, Binary Logic2/1
  Binary Logic1/1 -> Display3/1, Binary Logic2/2
  In1/1 -> Display/1, multiplier2/1

== system aes_impl_decrypt_smc/Round1/Subsystem8/Subsystem/Mixcolumn1 ==
  In1 : Inport
  In2 : Inport  Port=2
  In3 : Inport  Port=3
  In4 : Inport  Port=4
  Binary Logic : shlslibv1/Math Functions/Binary Logic  syn_binlog_exp=a^b  synBlockType=primitive  synLatency=0  synBlockId=13
  Binary Logic1 : shlslibv1/Math Functions/Binary Logic  syn_binlog_exp=a^b  synBlockType=primitive  synLatency=0  synBlockId=13
  Binary Logic2 : shlslibv1/Math Functions/Binary Logic  syn_binlog_exp=a^b  synBlockType=primitive  synLatency=0  synBlockId=13
  Display5 : Display
      settings: Format=hex (Stored Integer)
  Port Out : shlslibv1/Ports & Subsystems/Port Out  syn_capture=on  syn_register=on  synBlockType=port  synLatency=1  synBlockId=1
  multiplier2 : shlslibv1/Memories/ROM  syn_rom_vec=multiplier2  syn_rom_auto_wl=on  syn_out_wl=8  syn_out_fl=0  syn_out_dt=unsigned  syn_out_sat=on  syn_out_rnd=on  syn_en_port=off  synBlockType=primitive  synLatency=1  synBlockId=62  syn_dual_port=off
  multiplier4 : shlslibv1/Memories/ROM  syn_rom_vec=multiplier3  syn_rom_auto_wl=on  syn_out_wl=8  syn_out_fl=0  syn_out_dt=unsigned  syn_out_sat=on  syn_out_rnd=on  syn_en_port=off  synBlockType=primitive  synLatency=1  synBlockId=62  syn_dual_port=off
  Out1 : Outport
  wires:
  multiplier2/1 -> Binary Logic/2
  In2/1 -> multiplier2/1
  In4/1 -> Binary Logic1/2
  In1/1 -> Binary Logic/1
  multiplier4/1 -> Binary Logic1/1
  Binary Logic2/1 -> Port Out/1, Out1/1
  In3/1 -> multiplier4/1
  Port Out/1 -> Display5/1
  Binary Logic/1 -> Binary Logic2/1
  Binary Logic1/1 -> Binary Logic2/2

== system aes_impl_decrypt_smc/Round1/Subsystem8/Subsystem/Mixcolumn2 ==
  In1 : Inport
  In2 : Inport  Port=2
  In3 : Inport  Port=3
  In4 : Inport  Port=4
  Binary Logic : shlslibv1/Math Functions/Binary Logic  syn_binlog_exp=a^b  synBlockType=primitive  synLatency=0  synBlockId=13
  Binary Logic1 : shlslibv1/Math Functions/Binary Logic  syn_binlog_exp=a^b  synBlockType=primitive  synLatency=0  synBlockId=13
  Binary Logic2 : shlslibv1/Math Functions/Binary Logic  syn_binlog_exp=a^b  synBlockType=primitive  synLatency=0  synBlockId=13
  Display5 : Display
      settings: Format=hex (Stored Integer)
  Port Out : shlslibv1/Ports & Subsystems/Port Out  syn_capture=on  syn_register=on  synBlockType=port  synLatency=1  synBlockId=1
  multiplier2 : shlslibv1/Memories/ROM  syn_rom_vec=multiplier2  syn_rom_auto_wl=on  syn_out_wl=8  syn_out_fl=0  syn_out_dt=unsigned  syn_out_sat=on  syn_out_rnd=on  syn_en_port=off  synBlockType=primitive  synLatency=1  synBlockId=62  syn_dual_port=off
  multiplier3 : shlslibv1/Memories/ROM  syn_rom_vec=multiplier3  syn_rom_auto_wl=on  syn_out_wl=8  syn_out_fl=0  syn_out_dt=unsigned  syn_out_sat=on  syn_out_rnd=on  syn_en_port=off  synBlockType=primitive  synLatency=1  synBlockId=62  syn_dual_port=off
  Out1 : Outport
  wires:
  In1/1 -> Binary Logic/1
  Binary Logic2/1 -> Port Out/1, Out1/1
  In4/1 -> multiplier3/1
  In3/1 -> multiplier2/1
  In2/1 -> Binary Logic/2
  multiplier2/1 -> Binary Logic1/1
  multiplier3/1 -> Binary Logic1/2
  Binary Logic/1 -> Binary Logic2/1
  Binary Logic1/1 -> Binary Logic2/2
  Port Out/1 -> Display5/1

== system aes_impl_decrypt_smc/Round1/Subsystem8/Subsystem/Mixcolumn3 ==
  In1 : Inport
  In2 : Inport  Port=2
  In3 : Inport  Port=3
  In4 : Inport  Port=4
  Binary Logic : shlslibv1/Math Functions/Binary Logic  syn_binlog_exp=a^b  synBlockType=primitive  synLatency=0  synBlockId=13
  Binary Logic1 : shlslibv1/Math Functions/Binary Logic  syn_binlog_exp=a^b  synBlockType=primitive  synLatency=0  synBlockId=13
  Binary Logic2 : shlslibv1/Math Functions/Binary Logic  syn_binlog_exp=a^b  synBlockType=primitive  synLatency=0  synBlockId=13
  Display5 : Display
      settings: Format=hex (Stored Integer)
  Port Out : shlslibv1/Ports & Subsystems/Port Out  syn_capture=on  syn_register=on  synBlockType=port  synLatency=1  synBlockId=1
  multiplier1 : shlslibv1/Memories/ROM  syn_rom_vec=multiplier2  syn_rom_auto_wl=on  syn_out_wl=8  syn_out_fl=0  syn_out_dt=unsigned  syn_out_sat=on  syn_out_rnd=on  syn_en_port=off  synBlockType=primitive  synLatency=1  synBlockId=62  syn_dual_port=off
  multiplier4 : shlslibv1/Memories/ROM  syn_rom_vec=multiplier3  syn_rom_auto_wl=on  syn_out_wl=8  syn_out_fl=0  syn_out_dt=unsigned  syn_out_sat=on  syn_out_rnd=on  syn_en_port=off  synBlockType=primitive  synLatency=1  synBlockId=62  syn_dual_port=off
  Out1 : Outport
  wires:
  In2/1 -> Binary Logic/2
  multiplier1/1 -> Binary Logic1/2
  multiplier4/1 -> Binary Logic/1
  In3/1 -> Binary Logic1/1
  In1/1 -> multiplier4/1
  Binary Logic2/1 -> Port Out/1, Out1/1
  In4/1 -> multiplier1/1
  Port Out/1 -> Display5/1
  Binary Logic/1 -> Binary Logic2/1
  Binary Logic1/1 -> Binary Logic2/2

== system aes_impl_decrypt_smc/Round1/Subsystem8/Subsystem1/Mixcolumn ==
  In1 : Inport
  In2 : Inport  Port=2
  In3 : Inport  Port=3
  In4 : Inport  Port=4
  Binary Logic : shlslibv1/Math Functions/Binary Logic  syn_binlog_exp=a^b  synBlockType=primitive  synLatency=0  synBlockId=13
  Binary Logic1 : shlslibv1/Math Functions/Binary Logic  syn_binlog_exp=a^b  synBlockType=primitive  synLatency=0  synBlockId=13
  Binary Logic2 : shlslibv1/Math Functions/Binary Logic  syn_binlog_exp=a^b  synBlockType=primitive  synLatency=0  synBlockId=13
  Display5 : Display
      settings: Format=hex (Stored Integer)
  Port Out : shlslibv1/Ports & Subsystems/Port Out  syn_capture=on  syn_register=on  synBlockType=port  synLatency=1  synBlockId=1
  multiplier2 : shlslibv1/Memories/ROM  syn_rom_vec=multiplier2  syn_rom_auto_wl=on  syn_out_wl=8  syn_out_fl=0  syn_out_dt=unsigned  syn_out_sat=on  syn_out_rnd=on  syn_en_port=off  synBlockType=primitive  synLatency=1  synBlockId=62  syn_dual_port=off
  multiplier3 : shlslibv1/Memories/ROM  syn_rom_vec=multiplier3  syn_rom_auto_wl=on  syn_out_wl=8  syn_out_fl=0  syn_out_dt=unsigned  syn_out_sat=on  syn_out_rnd=on  syn_en_port=off  synBlockType=primitive  synLatency=1  synBlockId=62  syn_dual_port=off
  Out1 : Outport
  wires:
  multiplier3/1 -> Binary Logic/2
  In2/1 -> multiplier3/1
  In4/1 -> Binary Logic1/2
  multiplier2/1 -> Binary Logic/1
  In3/1 -> Binary Logic1/1
  Binary Logic2/1 -> Port Out/1, Out1/1
  In1/1 -> multiplier2/1
  Port Out/1 -> Display5/1
  Binary Logic/1 -> Binary Logic2/1
  Binary Logic1/1 -> Binary Logic2/2

== system aes_impl_decrypt_smc/Round1/Subsystem8/Subsystem1/Mixcolumn1 ==
  In1 : Inport
  In2 : Inport  Port=2
  In3 : Inport  Port=3
  In4 : Inport  Port=4
  Binary Logic : shlslibv1/Math Functions/Binary Logic  syn_binlog_exp=a^b  synBlockType=primitive  synLatency=0  synBlockId=13
  Binary Logic1 : shlslibv1/Math Functions/Binary Logic  syn_binlog_exp=a^b  synBlockType=primitive  synLatency=0  synBlockId=13
  Binary Logic2 : shlslibv1/Math Functions/Binary Logic  syn_binlog_exp=a^b  synBlockType=primitive  synLatency=0  synBlockId=13
  Display5 : Display
      settings: Format=hex (Stored Integer)
  Port Out : shlslibv1/Ports & Subsystems/Port Out  syn_capture=on  syn_register=on  synBlockType=port  synLatency=1  synBlockId=1
  multiplier2 : shlslibv1/Memories/ROM  syn_rom_vec=multiplier2  syn_rom_auto_wl=on  syn_out_wl=8  syn_out_fl=0  syn_out_dt=unsigned  syn_out_sat=on  syn_out_rnd=on  syn_en_port=off  synBlockType=primitive  synLatency=1  synBlockId=62  syn_dual_port=off
  multiplier4 : shlslibv1/Memories/ROM  syn_rom_vec=multiplier3  syn_rom_auto_wl=on  syn_out_wl=8  syn_out_fl=0  syn_out_dt=unsigned  syn_out_sat=on  syn_out_rnd=on  syn_en_port=off  synBlockType=primitive  synLatency=1  synBlockId=62  syn_dual_port=off
  Out1 : Outport
  wires:
  multiplier2/1 -> Binary Logic/2
  In2/1 -> multiplier2/1
  In4/1 -> Binary Logic1/2
  In1/1 -> Binary Logic/1
  multiplier4/1 -> Binary Logic1/1
  Binary Logic2/1 -> Port Out/1, Out1/1
  In3/1 -> multiplier4/1
  Port Out/1 -> Display5/1
  Binary Logic/1 -> Binary Logic2/1
  Binary Logic1/1 -> Binary Logic2/2

== system aes_impl_decrypt_smc/Round1/Subsystem8/Subsystem1/Mixcolumn2 ==
  In1 : Inport
  In2 : Inport  Port=2
  In3 : Inport  Port=3
  In4 : Inport  Port=4
  Binary Logic : shlslibv1/Math Functions/Binary Logic  syn_binlog_exp=a^b  synBlockType=primitive  synLatency=0  synBlockId=13
  Binary Logic1 : shlslibv1/Math Functions/Binary Logic  syn_binlog_exp=a^b  synBlockType=primitive  synLatency=0  synBlockId=13
  Binary Logic2 : shlslibv1/Math Functions/Binary Logic  syn_binlog_exp=a^b  synBlockType=primitive  synLatency=0  synBlockId=13
  Display5 : Display
      settings: Format=hex (Stored Integer)
  Port Out : shlslibv1/Ports & Subsystems/Port Out  syn_capture=on  syn_register=on  synBlockType=port  synLatency=1  synBlockId=1
  multiplier2 : shlslibv1/Memories/ROM  syn_rom_vec=multiplier2  syn_rom_auto_wl=on  syn_out_wl=8  syn_out_fl=0  syn_out_dt=unsigned  syn_out_sat=on  syn_out_rnd=on  syn_en_port=off  synBlockType=primitive  synLatency=1  synBlockId=62  syn_dual_port=off
  multiplier3 : shlslibv1/Memories/ROM  syn_rom_vec=multiplier3  syn_rom_auto_wl=on  syn_out_wl=8  syn_out_fl=0  syn_out_dt=unsigned  syn_out_sat=on  syn_out_rnd=on  syn_en_port=off  synBlockType=primitive  synLatency=1  synBlockId=62  syn_dual_port=off
  Out1 : Outport
  wires:
  In1/1 -> Binary Logic/1
  Binary Logic2/1 -> Port Out/1, Out1/1
  In4/1 -> multiplier3/1
  In3/1 -> multiplier2/1
  In2/1 -> Binary Logic/2
  multiplier2/1 -> Binary Logic1/1
  multiplier3/1 -> Binary Logic1/2
  Binary Logic/1 -> Binary Logic2/1
  Binary Logic1/1 -> Binary Logic2/2
  Port Out/1 -> Display5/1

== system aes_impl_decrypt_smc/Round1/Subsystem8/Subsystem1/Mixcolumn3 ==
  In1 : Inport
  In2 : Inport  Port=2
  In3 : Inport  Port=3
  In4 : Inport  Port=4
  Binary Logic : shlslibv1/Math Functions/Binary Logic  syn_binlog_exp=a^b  synBlockType=primitive  synLatency=0  synBlockId=13
  Binary Logic1 : shlslibv1/Math Functions/Binary Logic  syn_binlog_exp=a^b  synBlockType=primitive  synLatency=0  synBlockId=13
  Binary Logic2 : shlslibv1/Math Functions/Binary Logic  syn_binlog_exp=a^b  synBlockType=primitive  synLatency=0  synBlockId=13
  Display5 : Display
      settings: Format=hex (Stored Integer)
  Port Out : shlslibv1/Ports & Subsystems/Port Out  syn_capture=on  syn_register=on  synBlockType=port  synLatency=1  synBlockId=1
  multiplier1 : shlslibv1/Memories/ROM  syn_rom_vec=multiplier2  syn_rom_auto_wl=on  syn_out_wl=8  syn_out_fl=0  syn_out_dt=unsigned  syn_out_sat=on  syn_out_rnd=on  syn_en_port=off  synBlockType=primitive  synLatency=1  synBlockId=62  syn_dual_port=off
  multiplier4 : shlslibv1/Memories/ROM  syn_rom_vec=multiplier3  syn_rom_auto_wl=on  syn_out_wl=8  syn_out_fl=0  syn_out_dt=unsigned  syn_out_sat=on  syn_out_rnd=on  syn_en_port=off  synBlockType=primitive  synLatency=1  synBlockId=62  syn_dual_port=off
  Out1 : Outport
  wires:
  In2/1 -> Binary Logic/2
  multiplier1/1 -> Binary Logic1/2
  multiplier4/1 -> Binary Logic/1
  In3/1 -> Binary Logic1/1
  In1/1 -> multiplier4/1
  Binary Logic2/1 -> Port Out/1, Out1/1
  In4/1 -> multiplier1/1
  Port Out/1 -> Display5/1
  Binary Logic/1 -> Binary Logic2/1
  Binary Logic1/1 -> Binary Logic2/2
